simulink model "labo3_redresseur_monophase_point_milieu"  (R2018a)
settings: Solver=ode15s  StartTime=0.0  StopTime=0.1  RelTol=1e-3
libraries: powerlib x10
settings Model: Creator=deniz  LastModifiedBy=deniz

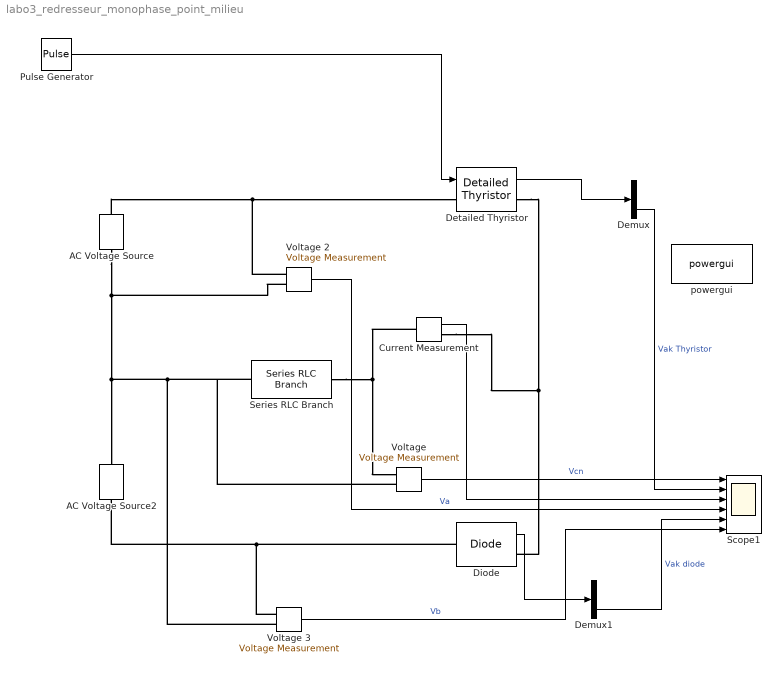
== system labo3_redresseur_monophase_point_milieu ==
  AC Voltage Source : powerlib/Electrical Sources/AC Voltage Source  Amplitude=170  Phase=0  Frequency=60  SampleTime=0  Measurements=None  BusType=swing  Pref=10e3  Qref=0  Qmin=-inf  Qmax=+inf
  AC Voltage Source2 : powerlib/Electrical Sources/AC Voltage Source  Amplitude=170  Phase=0  Frequency=60  SampleTime=0  Measurements=None  BusType=swing  Pref=10e3  Qref=0  Qmin=-inf  Qmax=+inf
  Current Measurement : powerlib/Measurements/Current Measurement  PhasorSimulation=off  OutputType=Complex  PSBequivalent=0
  Demux : Demux  Outputs=2
  Demux1 : Demux  Outputs=2
  Detailed Thyristor : powerlib/Power Electronics/Detailed Thyristor  Ron=0.1  Lon=10e-6  Vf=0.8  IL=0.3  Tq=100e-6  IC=0  Rs=1000  Cs=1e-7  Measurements=on
      settings: SourceProductName=Simscape Power Systems  SourceProductBaseCode=PS
  Diode : powerlib/Power Electronics/Diode  Ron=0.001  Lon=0  Vf=0.8  IC=0  UseSnubber=0  Rs=500  Cs=250e-9  Measurements=on
  Pulse Generator : DiscretePulseGenerator  PulseType=Time based  Period=1/60  PulseWidth=5  PhaseDelay=(1/60)*(90/360)
  Scope1 : Scope  NumInputPorts=6
  Series RLC Branch : powerlib/Elements/Series RLC Branch  LConnTagsString=__new0  RConnTagsString=__new0  BranchType=RLC  Resistance=24  Inductance=0.050  SetiL0=off  InitialCurrent=0  Capacitance=inf  Setx0=off  InitialVoltage=0  Measurements=None
  "Voltage " : powerlib/Measurements/Voltage Measurement  PhasorSimulation=off  OutputType=Complex  PSBequivalent=0
  Voltage 2 : powerlib/Measurements/Voltage Measurement  PhasorSimulation=off  OutputType=Complex  PSBequivalent=0
  Voltage 3 : powerlib/Measurements/Voltage Measurement  PhasorSimulation=off  OutputType=Complex  PSBequivalent=0
  powergui : powerlib/powergui  Priority=1  SimulationMode=Continuous  SampleTime=50e-6  frequency=60  Iterations=50  frequencyindice=60  Pbase=100e6  ErrMax=1e-4  UnitsV=kV  UnitsW=MW  buscounter=0  FunctionMessages=off  echomessages=off  EnableUseOfTLC=off  CurrentSourceSwitches=off  DisableSnubberDevices=off  DisableRonSwitches=off  DisableVfSwitches=off  DisplayEquations=off  SolverType=Tustin/Backward Euler (TBE)  Interpol=off  ExternalGateDelay=off  methode=off  Ts=100  x0status=blocks  SPID=off  SwTol=0  HookPort=off  RestoreLinks=warning  ResistiveCurrentMeasurement=off  Frange=[0:2:500]  Ylog=off  Xlog=on  ShowGrid=off  save=off  variable=ZData  structure=0  ZoomFFT=off  StartTime=0.0  cycles=1  DisplayStyle=1  fundamental=60  FreqAxis=off  MaxFrequency=1000  frequencyindicesteady=1  RmsSteady=1  display=off
  wires:
  Pulse Generator/1 -> Detailed Thyristor/1
  "Voltage "/1 -> Scope1/1  "Vcn"
  Detailed Thyristor/1 -> Demux/1
  Demux/2 -> Scope1/2  "Vak Thyristor"
  Diode/1 -> Demux1/1
  Demux1/2 -> Scope1/5  "Vak diode"
  Voltage 2/1 -> Scope1/4  "Va"
  Voltage 3/1 -> Scope1/6  "Vb"
  Current Measurement/1 -> Scope1/3
  connections:
  AC Voltage Source/RConn1 -- Voltage 2/LConn1 -- Detailed Thyristor/LConn1
  Series RLC Branch/RConn1 -- Current Measurement/LConn1 -- "Voltage "/LConn1
  AC Voltage Source/LConn1 -- Voltage 2/LConn2 -- Voltage 3/LConn2 -- "Voltage "/LConn2 -- Series RLC Branch/LConn1 -- AC Voltage Source2/RConn1
  Diode/LConn1 -- Voltage 3/LConn1 -- AC Voltage Source2/LConn1
  Detailed Thyristor/RConn1 -- Current Measurement/RConn1 -- Diode/RConn1
